simulink model "submission_hump"  (R2021b)
settings: Solver=VariableStepAuto  StartTime=0.0  StopTime=10.0  RelTol=1e-3
settings Model: Creator=matth  LastModifiedBy=matth

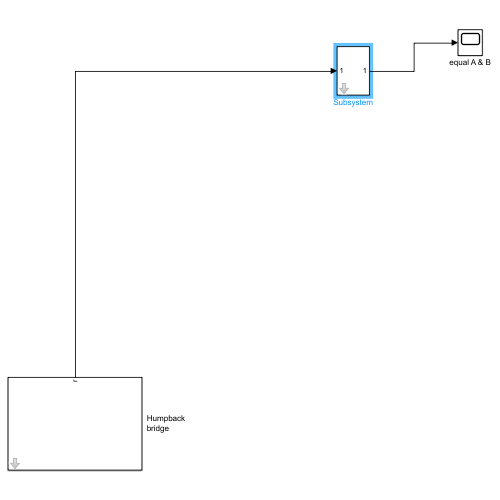
[thumbnail: Simulink's stored preview of the top-level diagram]
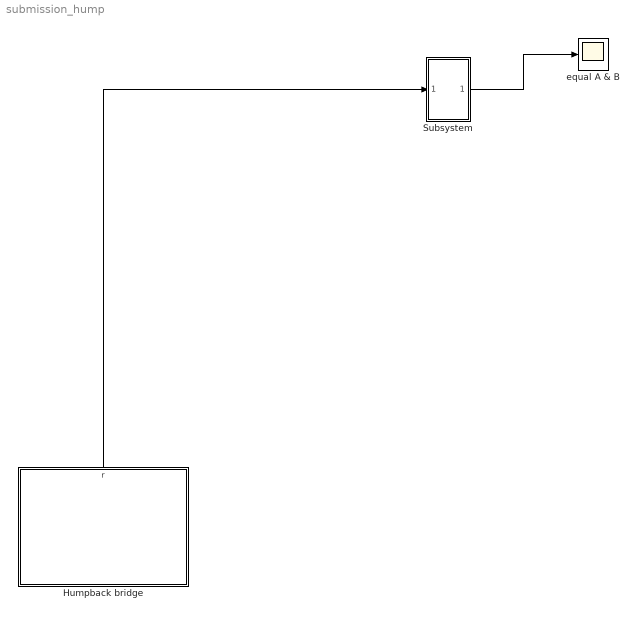
== system submission_hump ==
  Humpback bridge : Subsystem  mask{h=2, L=20, v=20}
      mask prompts: h "humpback height (m)"; L "humpback length (m)"; v "vehicle speed (m/s)"
  Subsystem : Subsystem  mask{m1=500, m2=20, a=1, b=1, Ib=600, ks=20000, kss=4000000, cs=600, css=12000, x0=0.2, g=9.81, kt=140000}
      mask prompts: m1 "mass body"; m2 "mass wheel"; a "length front"; b "length rear"; Ib "Moment of inertia"; ks "stiffness suspension"; kss "spring hardening"; cs "damping"; css "damping extention"; g "gravitation acceleration"; kt "stiffness tyre"
  equal A & B : Scope
  wires:
  Humpback bridge/1(r) -> Subsystem/1(In1)
  Subsystem/1(Out1) -> equal A & B/1

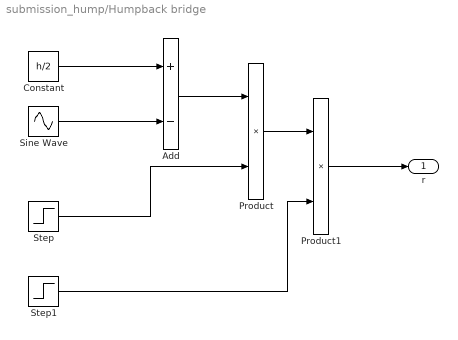
== system submission_hump/Humpback bridge ==
  Add : Sum  Inputs=+-
  Constant : Constant  Value=h/2
  Product : Product
  Product1 : Product
  Sine Wave : Sin  Amplitude=h/2  Frequency=2*pi*v/L  Phase=pi/2  SampleTime=0
  Step : Step  Time=2*L/v  SampleTime=0
  Step1 : Step  Time=3*L/v  Before=1  After=0  SampleTime=0
  r : Outport
  wires:
  Constant/1 -> Add/1
  Sine Wave/1 -> Add/2
  Add/1 -> Product/1
  Step/1 -> Product/2
  Product/1 -> Product1/1
  Step1/1 -> Product1/2
  Product1/1 -> r/1

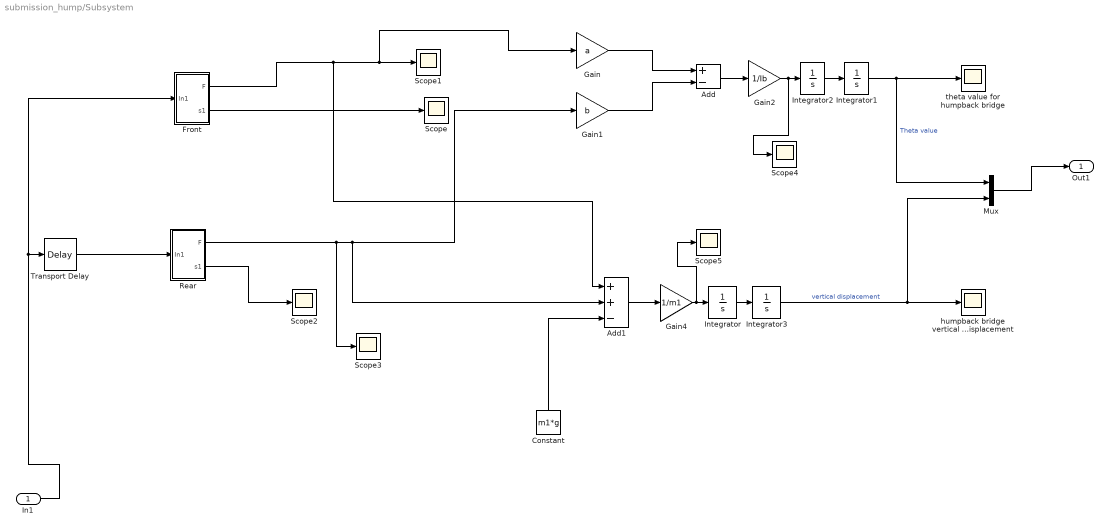
== system submission_hump/Subsystem ==
  In1 : Inport
  Add : Sum  Inputs=+-
  Add1 : Sum  Inputs=++-
  Constant : Constant  Value=m1*g
  "Front " : Subsystem
  Gain : Gain  Gain=a
  Gain1 : Gain  Gain=b
  Gain2 : Gain  Gain=1/Ib
  Gain4 : Gain  Gain=1/m1
  Integrator{,1..3} (4 alike) : Integrator
  Mux : Mux  Inputs=2
  Rear : Subsystem
  Scope{,1..5} (6 alike) : Scope
  Transport Delay : TransportDelay  DelayTime=0.1325  FixedBuffer=on
  humpback bridge vertical displacement : Scope
  theta value for humpback bridge : Scope
  Out1 : Outport
  wires:
  Add/1 -> Gain2/1
  "Front "/1(F) -> Add1/1, Gain/1, Scope1/1
  Gain2/1 -> Scope4/1, Integrator2/1
  Rear/2(s1) -> Scope2/1
  Constant/1 -> Add1/3
  In1/1 -> "Front "/1(In1), Transport Delay/1
  Transport Delay/1 -> Rear/1(In1)
  Rear/1(F) -> Scope3/1, Add1/2, Gain1/1
  Gain/1 -> Add/1
  "Front "/2(s1) -> Scope/1
  Integrator1/1 -> Mux/1, theta value for humpback bridge/1  "Theta value"
  Add1/1 -> Gain4/1
  Gain4/1 -> Scope5/1, Integrator/1
  Gain1/1 -> Add/2
  Integrator3/1 -> Mux/2, humpback bridge vertical displacement/1  "vertical displacement"
  Integrator2/1 -> Integrator1/1
  Integrator/1 -> Integrator3/1
  Mux/1 -> Out1/1

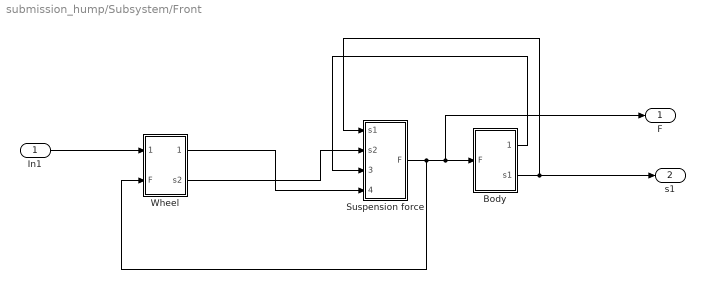
== system submission_hump/Subsystem/Front  ==
  In1 : Inport
  Body : Subsystem
  Suspension force : Subsystem
  Wheel : Subsystem
  F : Outport
  s1 : Outport  Port=2
  wires:
  Body/1(S1dot) -> Suspension force/3(S1dot)
  Wheel/2(s2) -> Suspension force/2(s2)
  Body/2(s1) -> s1/1, Suspension force/1(s1)
  Suspension force/1(F) -> Wheel/2(F), F/1, Body/1(F)
  Wheel/1(s2dot) -> Suspension force/4(s2dot)
  In1/1 -> Wheel/1(In1)

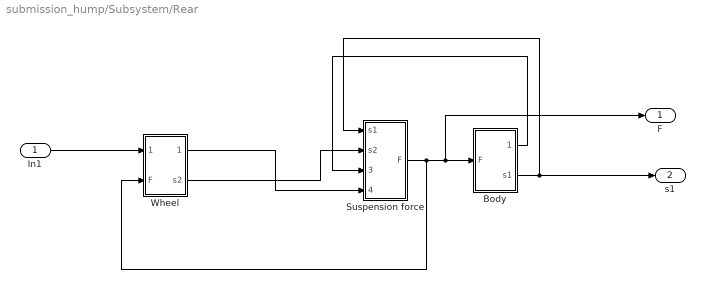
== system submission_hump/Subsystem/Rear ==
  In1 : Inport
  Body : Subsystem
  Suspension force : Subsystem
  Wheel : Subsystem
  F : Outport
  s1 : Outport  Port=2
  wires:
  Body/1(S1dot) -> Suspension force/3(S1dot)
  Wheel/2(s2) -> Suspension force/2(s2)
  Body/2(s1) -> s1/1, Suspension force/1(s1)
  Suspension force/1(F) -> Wheel/2(F), F/1, Body/1(F)
  Wheel/1(s2dot) -> Suspension force/4(s2dot)
  In1/1 -> Wheel/1(In1)

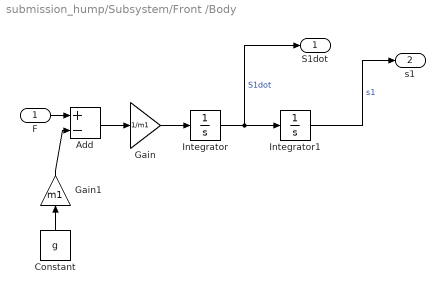
== system submission_hump/Subsystem/Front /Body ==
  F : Inport
  Add : Sum  Inputs=+-
  Constant : Constant  Value=g
  Gain : Gain  Gain=1/m1
  Gain1 : Gain  Gain=m1
  Integrator : Integrator
  Integrator1 : Integrator
  S1dot : Outport
  s1 : Outport  Port=2
  wires:
  Gain1/1 -> Add/2
  Add/1 -> Gain/1
  Constant/1 -> Gain1/1
  Gain/1 -> Integrator/1
  Integrator1/1 -> s1/1  "s1"
  Integrator/1 -> S1dot/1, Integrator1/1  "S1dot"
  F/1 -> Add/1

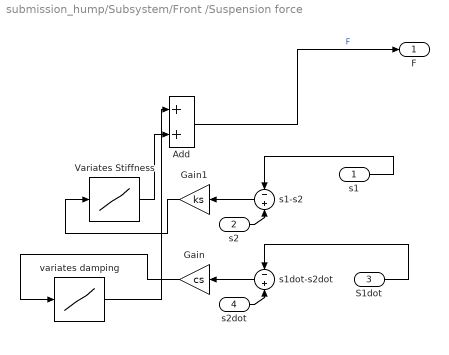
== system submission_hump/Subsystem/Front /Suspension force ==
  s1 : Inport
  s2 : Inport  Port=2
  S1dot : Inport  Port=3
  s2dot : Inport  Port=4
  Add : Sum
  Gain : Gain  Gain=cs
  Gain1 : Gain  Gain=ks
  Variates Stiffness : Lookup_n-D  NumberOfTableDimensions=1  BreakpointsForDimension1=[-2*x0, -x0, x0, 2*x0]  Table=[-(ks+kss)*x0, -ks*x0, ks*x0, (ks+kss)*x0]  InternalRulePriority=Speed  RndMeth=Simplest  InputSameDT=on
  s1-s2 : Sum  Inputs=-+
  s1dot-s2dot : Sum  Inputs=-+
  variates damping : Lookup_n-D  NumberOfTableDimensions=1  BreakpointsForDimension1=[-2*x0, -x0, x0, 2*x0]  Table=[-(cs+css)*x0, -cs*x0, cs*x0, (cs+css)*x0]  InternalRulePriority=Speed  RndMeth=Simplest  InputSameDT=on
  F : Outport
  wires:
  Gain1/1 -> Variates Stiffness/1
  variates damping/1 -> Add/1
  S1dot/1 -> s1dot-s2dot/1
  s1dot-s2dot/1 -> Gain/1
  s1-s2/1 -> Gain1/1
  Gain/1 -> variates damping/1
  Add/1 -> F/1  "F"
  Variates Stiffness/1 -> Add/2
  s2dot/1 -> s1dot-s2dot/2
  s1/1 -> s1-s2/1
  s2/1 -> s1-s2/2

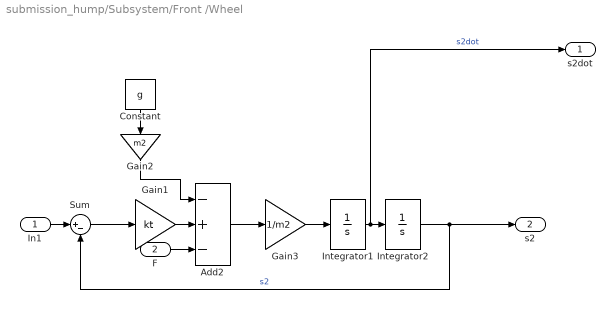
== system submission_hump/Subsystem/Front /Wheel ==
  In1 : Inport
  F : Inport  Port=2
  Add2 : Sum  Inputs=-+-
  Constant : Constant  Value=g
  Gain1 : Gain  Gain=kt
  Gain2 : Gain  Gain=m2
  Gain3 : Gain  Gain=1/m2
  Integrator1 : Integrator
  Integrator2 : Integrator
  Sum : Sum  Inputs=|+-
  s2dot : Outport
  s2 : Outport  Port=2
  wires:
  F/1 -> Add2/3
  Gain2/1 -> Add2/1
  Integrator1/1 -> s2dot/1, Integrator2/1  "s2dot"
  Add2/1 -> Gain3/1
  Gain3/1 -> Integrator1/1
  Sum/1 -> Gain1/1
  Gain1/1 -> Add2/2
  Constant/1 -> Gain2/1
  Integrator2/1 -> Sum/2, s2/1  "s2"
  In1/1 -> Sum/1

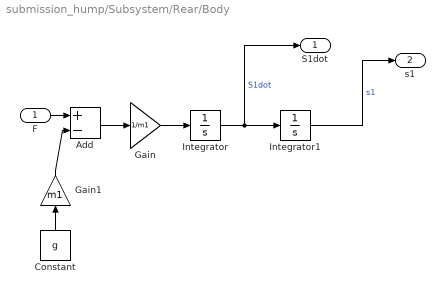
== system submission_hump/Subsystem/Rear/Body ==
  F : Inport
  Add : Sum  Inputs=+-
  Constant : Constant  Value=g
  Gain : Gain  Gain=1/m1
  Gain1 : Gain  Gain=m1
  Integrator : Integrator
  Integrator1 : Integrator
  S1dot : Outport
  s1 : Outport  Port=2
  wires:
  Gain1/1 -> Add/2
  Add/1 -> Gain/1
  Constant/1 -> Gain1/1
  Gain/1 -> Integrator/1
  Integrator1/1 -> s1/1  "s1"
  Integrator/1 -> S1dot/1, Integrator1/1  "S1dot"
  F/1 -> Add/1

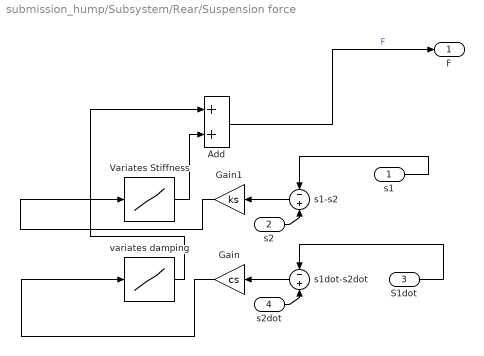
== system submission_hump/Subsystem/Rear/Suspension force ==
  s1 : Inport
  s2 : Inport  Port=2
  S1dot : Inport  Port=3
  s2dot : Inport  Port=4
  Add : Sum
  Gain : Gain  Gain=cs
  Gain1 : Gain  Gain=ks
  Variates Stiffness : Lookup_n-D  NumberOfTableDimensions=1  BreakpointsForDimension1=[-2*x0, -x0, x0, 2*x0]  Table=[-(ks+kss)*x0, -ks*x0, ks*x0, (ks+kss)*x0]  InternalRulePriority=Speed  RndMeth=Simplest  InputSameDT=on
  s1-s2 : Sum  Inputs=-+
  s1dot-s2dot : Sum  Inputs=-+
  variates damping : Lookup_n-D  NumberOfTableDimensions=1  BreakpointsForDimension1=[-2*x0, -x0, x0, 2*x0]  Table=[-(cs+css)*x0, -cs*x0, cs*x0, (cs+css)*x0]  InternalRulePriority=Speed  RndMeth=Simplest  InputSameDT=on
  F : Outport
  wires:
  Gain1/1 -> Variates Stiffness/1
  variates damping/1 -> Add/1
  S1dot/1 -> s1dot-s2dot/1
  s1dot-s2dot/1 -> Gain/1
  s1-s2/1 -> Gain1/1
  Gain/1 -> variates damping/1
  Add/1 -> F/1  "F"
  Variates Stiffness/1 -> Add/2
  s2dot/1 -> s1dot-s2dot/2
  s1/1 -> s1-s2/1
  s2/1 -> s1-s2/2

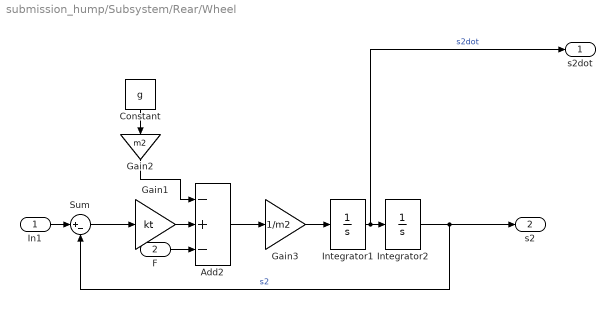
== system submission_hump/Subsystem/Rear/Wheel ==
  In1 : Inport
  F : Inport  Port=2
  Add2 : Sum  Inputs=-+-
  Constant : Constant  Value=g
  Gain1 : Gain  Gain=kt
  Gain2 : Gain  Gain=m2
  Gain3 : Gain  Gain=1/m2
  Integrator1 : Integrator
  Integrator2 : Integrator
  Sum : Sum  Inputs=|+-
  s2dot : Outport
  s2 : Outport  Port=2
  wires:
  F/1 -> Add2/3
  Gain2/1 -> Add2/1
  Integrator1/1 -> s2dot/1, Integrator2/1  "s2dot"
  Add2/1 -> Gain3/1
  Gain3/1 -> Integrator1/1
  Sum/1 -> Gain1/1
  Gain1/1 -> Add2/2
  Constant/1 -> Gain2/1
  Integrator2/1 -> Sum/2, s2/1  "s2"
  In1/1 -> Sum/1
